simulink model "VSC_GF_2bus_nonlinear"  (R2021b)
settings: Solver=ode45  StartTime=0.0  StopTime=Tsim  FixedStep=10e-6  RelTol=1e-6  EnableMultiTasking=on
values from neighbouring files (symbols this model uses):
  angle_g1_fnl = 0.0    (= 0)    [params_pu.m]
  angle_g1_init = 0.0    (= 0)    [params_pu.m]
  Cac_n1 = 0.15/wb_n1    (= 0.000477464829276)    [params_pu.m]
  k_droop_u_n1 = (0.02/0.3)*(sqrt(2)/sqrt(3))    [params_pu.m]
  ki_pll1 = kp_pll1/tau_pll_n1    [params_pu.m]
  ki_vac_n1 = 42.05*(Vb_n1/Ib_n1)    (= 7.28000181818)    [params_pu.m]
  kp_pll1 = xi_pll_n1*2*omega_pll_n1/(sqrt(2)/sqrt(3))    [params_pu.m]
  kp_vac_n1 = 4.789*(Vb_n1/Ib_n1)    (= 0.829106509091)    [params_pu.m]
  Lc_n1 = 0.15/wb_n1    (= 0.000477464829276)    [params_pu.m]
  Lg_n1 = Xg_n1/wb_n1    [params_pu.m]
  Lg_n2 = imag(Zg_n2)/wb_n1    [params_pu.m]
  magnitud_delay = 1e-5    (= 1e-05)    [params_pu.m]
  P_ref_n1 = 0.5    [params_pu.m]
  plots_step = 10e-6    (= 1e-05)    [params_pu.m]
  Q_ref_n1 = 0.1    [params_pu.m]
  Rac_n1 = 1/(3*10*wb_n1*Cac_n1)    (= 0.222222222222)    [params_pu.m]
  Rg_n1 = Rg_n1/Zb_n1    [params_pu.m]
  Rg_n2 = real(Zg_n2)    [params_pu.m]
  Rseries_n1 = 5e-4/Zb_n1    (= 0.00288804872926)    [params_pu.m]
  T_stp = Tsim/2    (= 2)    [params_pu.m]
  tau_droop_f = 1/50    (= 0.02)    [params_pu.m]
  tau_droop_u = 1/50    (= 0.02)    [params_pu.m]
  tau_ig = 0.1e-3    (= 0.0001)    [params_pu.m]
  tau_u = 0.1e-3    (= 0.0001)    [params_pu.m]
  Vb_dc_n1 = 2e3    (= 2000)    [params_pu.m]
  Vb_n1 = 0.69e3    (= 690)    [params_pu.m]
  Vdcref_n1 = Vb_dc_n1    (= 2000)    [params_pu.m]
  Vpeak_g1_fnl = 0.98*(sqrt(2)/sqrt(3))    [params_pu.m]
  Vpeak_g1_init = 1*(sqrt(2)/sqrt(3))    [params_pu.m]
  Vpeak_n1 = Vb_n1/sqrt(3)*sqrt(2)    [params_pu.m]
  wb_n1 = 2*pi*fb_n1    (= 314.159265359)    [params_pu.m]
undefined symbols (not defined in the file or in its folder): Cac, DRload, Ib_vsc, is_dc0, is_qc0, k_droop_f, ki_s, ki_vac, kp_s, kp_vac, Lc, Lf, Ltr, P, Rac, Rc, Rtr, Sb, T_load, tstep, u_dc0, u_q0, u_qc0, Vb_vsc, vc_dc0, vc_qc0, wb, Zb
libraries: spsSeriesRLCBranchLib x42, spsParallelRLCBranchLib x21, spsControlledVoltageSourceLib x14, spsCurrentMeasurementLib x14, spsGroundLib x10, slpidlib x9, spsVoltageMeasurementLib x6, spsThreePhaseVIMeasurementLib x2, spsPower3phInstantaneousLib x2, spsThreePhaseBreakerLib x2, spsControlledCurrentSourceLib x2, eeTransforms x1
(part 1 of 3)
settings Model: ExtModeTrigDuration=100  Creator=Enric  LastModifiedBy=CITCEA
settings SolverCC: SolverJacobianMethodControl=FullPerturbation  AlgebraicLoopSolver=TrustRegion
settings DataIOCC: LimitDataPoints=on  SaveOutput=off  ReturnWorkspaceOutputs=off  StateSaveName=tmp_raccel_xout  SignalLoggingName=tmp_raccel_logsout
settings OptimizationCC: EfficientMapNaN2IntZero=off  LifeSpan=inf
settings DebuggingCC: AllowSymbolicDim=off  SFUnexpectedBacktrackingDiag=warning  SFNoUnconditionalDefaultTransitionDiag=warning  SFExecutionAtInitializationDiag=none  SFMachineParentedDataDiag=warning  ArithmeticOperatorsInVariantConditions=warning
settings HardwareCC: TargetBitPerPointer=64  TargetBitPerSizeT=64  TargetBitPerPtrDiffT=64  TargetLongLongMode=on  TargetIntDivRoundTo=Zero  TargetEndianess=LittleEndian  TargetWordSize=64  TargetHWDeviceType=MATLAB Host  ProdEqTarget=off
settings ModelReferenceCC: PropagateSignalLabelsOutOfModel=off
settings SFSimCC: SimUseLocalCustomCode=off  CustomCodeUndefinedFunction=UseInterfaceOnly
settings RTWCC: SystemTargetFile=raccel.tlc  TemplateMakefile=raccel_default_tmf  RTWVerbose=off  RTWUseLocalCustomCode=off  RTWUseSimCustomCode=on
settings CodeAppCC: GenerateComments=off  MaxIdLength=128  MangleLength=10  SimulinkBlockComments=off
settings RaccelTargetCC: ENABLE_SLEXEC_SSBRIDGE=0  RTWCAPISignals=off  RTWCAPIParams=on  RTWCAPIRootIO=off
settings ConfigComp: CovMetricSettings=dw  CovSaveCumulativeToWorkspaceVar=on  CovSaveSingleToWorkspaceVar=on  CovExternalEMLEnable=off
settings SimscapeCC: SimscapeNormalizeSystem=off

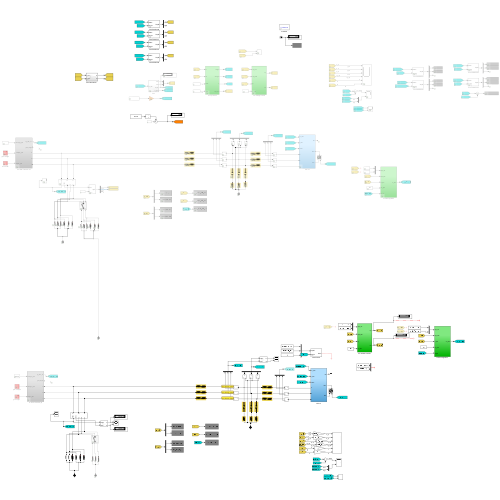
[thumbnail: Simulink's stored preview of the top-level diagram]
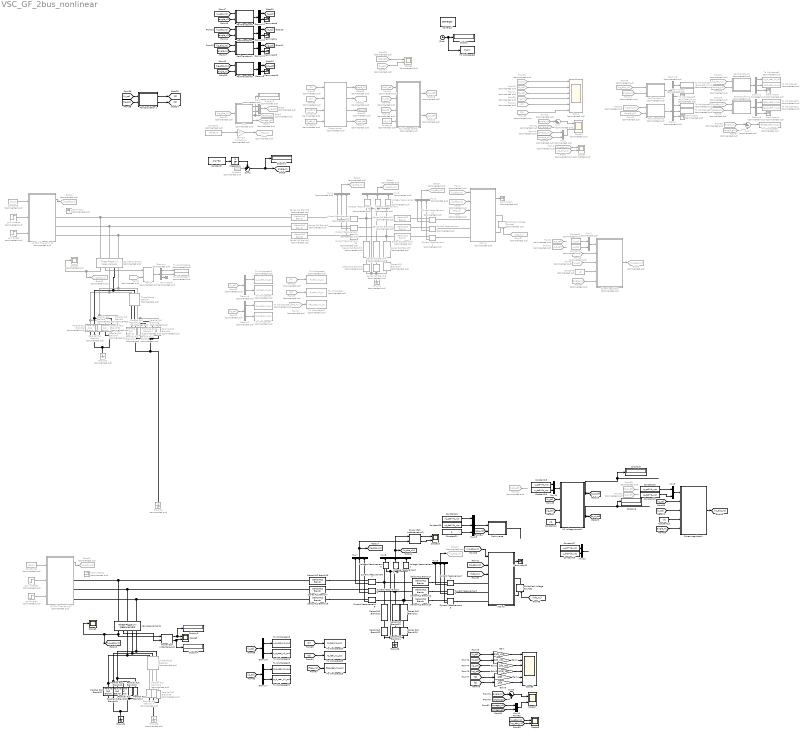
== system VSC_GF_2bus_nonlinear ==
  AC Grid Thevenin g1 : Subsystem  Commented=on
  AC Grid Thevenin g2 : Subsystem  Commented=on
  AC voltage control : Subsystem  Commented=on
  AC voltage control1 : Subsystem
  Clock : Clock
  Constant : Constant  Commented=on  Value=-pi/2
  Constant1 : Constant  Commented=on  Value=Vdcref_n1
  Constant10 : Constant  Value=is_qc0*Ib_vsc
  Constant11 : Constant  Commented=on  Value=wb_n1
  Constant12 : Constant  Value=wb
  Constant13 : Constant  Value=is_dc0*Ib_vsc
  Constant14 : Constant  Value=wb
  Constant15 : Constant  Value=u_qc0*Vb_vsc
  Constant16 : Constant  Value=u_dc0*Vb_vsc
  Constant17 : Constant  Value=u_qc0*Vb_vsc
  Constant18 : Constant  Value=u_dc0*Vb_vsc
  Constant19 : Constant  Value=vc_qc0*Vb_vsc
  Constant2 : Constant  Commented=on  Value=is_qc0
  Constant20 : Constant  Value=vc_dc0*Vb_vsc
  Constant21 : Constant  Value=0
  Constant3 : Constant  Commented=on  Value=P_ref_n1
  Constant4 : Constant  Commented=on  Value=wb_n1
  Constant5 : Constant  Commented=on  Value=wb_n1
  Constant6 : Constant  Commented=on  Value=wb
  Constant7 : Constant  Commented=on  Value=Q_ref_n1
  Constant8 : Constant  Commented=on  Value=is_dc0
  Constant9 : Constant  Value=2*pi*50
  Controlled Voltage Source1 : spsControlledVoltageSourceLib/Controlled Voltage Source  Commented=on  Initialize=off  Source_Type=DC  Amplitude=Vdcref_n1  Phase=0  Frequency=0  Measurements=None
  Controlled Voltage Source2 : spsControlledVoltageSourceLib/Controlled Voltage Source  Initialize=off  Source_Type=DC  Amplitude=Vdcref_n1  Phase=0  Frequency=0  Measurements=None
  Current Measurement{1..2,10,20..21,25} (6 alike) : spsCurrentMeasurementLib/Current Measurement  Commented=on  PhasorSimulation=off  OutputType=Complex  PSBequivalent=0
  Current Measurement{3..8} (6 alike) : spsCurrentMeasurementLib/Current Measurement  PhasorSimulation=off  OutputType=Complex  PSBequivalent=0
  Current regulator : Subsystem  Commented=on
  Current regulator1 : Subsystem
  Demux{,2,4,6,8} (5 alike) : Demux  Commented=on  Outputs=3
  Demux1 : Demux  Commented=on  Outputs=2
  Demux{5,7,9..11,13} (6 alike) : Demux  Outputs=2
  Demux3 : Demux  Commented=on  Outputs=2
  Display{,1,3..6} (6 alike) : Display
  Display2 : Display  Commented=on
  Droop control : Subsystem  Commented=on
  From : From  Commented=on  GotoTag=Vdc_n1
  From1 : From  Commented=on  GotoTag=vc_abc_n1
  From{10,22,34,56} (4 alike) : From  Commented=on  GotoTag=angle_g1
  From{3,11,23,35,52} (5 alike) : From  Commented=on  GotoTag=angle_n1  TagVisibility=global
  From12 : From  Commented=on  GotoTag=P
  From15 : From  Commented=on  GotoTag=is_qd
  From18 : From  Commented=on  GotoTag=is_qd
  From19 : From  Commented=on  GotoTag=is_d_ref
  From2 : From  Commented=on  GotoTag=theta_g
  From{8,20,30,44,46} (5 alike) : From  Commented=on  GotoTag=u_qd
  From21 : From  Commented=on  GotoTag=ig_qd
  From24 : From  Commented=on  GotoTag=P
  From25 : From  Commented=on  GotoTag=Q
  From26 : From  Commented=on  GotoTag=ig_abc_n1
  From27 : From  Commented=on  GotoTag=is_qd
  From28 : From  Commented=on  GotoTag=P
  From29 : From  Commented=on  GotoTag=Q
  From{7,31..32,43} (4 alike) : From  Commented=on  GotoTag=vg_abc_n1
  From33 : From  Commented=on  GotoTag=vg_qd
  From37 : From  Commented=on  GotoTag=Vdc_n1
  From39 : From  Commented=on  GotoTag=vqd_ref
  From4 : From  Commented=on  GotoTag=freq_n1
  From40 : From  Commented=on  GotoTag=omega_g1
  From41 : From  Commented=on  GotoTag=omega_n1
  From49 : From  Commented=on  GotoTag=ig_qd
  From5 : From  Commented=on  GotoTag=is_q_ref
  From51 : From  Commented=on  GotoTag=ig_abc_n1
  From54 : From  Commented=on  GotoTag=vqd_ref
  From55 : From  Commented=on  GotoTag=Q
  From6 : From  Commented=on  GotoTag=u_abc_n1
  From60 : From  Commented=on  GotoTag=is_d_ref
  From61 : From  Commented=on  GotoTag=vqd_ref
  From68 : From  Commented=on  GotoTag=is_q_ref
  From9 : From  Commented=on  GotoTag=is_abc_n1
  Gain : Gain  Gain=1/Vb_vsc
  Gain1 : Gain  Gain=1/Ib_vsc
  Gain10 : Gain  Commented=on  Gain=1/Vb_dc_n1
  Gain2 : Gain  Gain=1/Ib_vsc
  Gain3 : Gain  Gain=1/Vb_vsc
  Gain4 : Gain  Gain=1/Sb
  Gain5 : Gain  Gain=1/Sb
  Goto : Goto  Commented=on  GotoTag=Vdc_n1
  Goto1 : Goto  Commented=on  GotoTag=u_abc_n1
  Goto12 : Goto  Commented=on  GotoTag=vg_abc_n1
  Goto16 : Goto  Commented=on  GotoTag=vg_abc_n1
  Goto18 : Goto  Commented=on  GotoTag=is_q_ref
  Goto19 : Goto  Commented=on  GotoTag=is_d_ref
  Goto2 : Goto  Commented=on  GotoTag=vg_abc_n1
  Goto21 : Goto  Commented=on  GotoTag=omega_n1
  Goto22 : Goto  Commented=on  GotoTag=freq_n1
  Goto25 : Goto  Commented=on  GotoTag=vqd_ref
  Goto27 : Goto  Commented=on  GotoTag=is_abc_n1
  Goto3 : Goto  Commented=on  GotoTag=ig_abc_n1
  Goto4 : Goto  Commented=on  GotoTag=angle_g1
  Goto59 : Goto  Commented=on  GotoTag=angle_n1
  Goto6 : Goto  Commented=on  GotoTag=vc_abc_n1
  Goto7 : Goto  Commented=on  GotoTag=omega_g1
  Goto8 : Goto  Commented=on  GotoTag=vg_qd
  Goto9 : Goto  Commented=on  GotoTag=is_abc_n1
  Ground{,1..2,5} (4 alike) : spsGroundLib/Ground  Commented=on  LConnTagsString=a
  Ground3 : spsGroundLib/Ground  LConnTagsString=a
  Ground4 : spsGroundLib/Ground  LConnTagsString=a
  Icg measurement : spsThreePhaseVIMeasurementLib/Three-Phase V-I Measurement  Commented=on  VoltageMeasurement=phase-to-ground  SetLabelV=off  LabelV=Uabc  Vpu=off  VpuLL=off  CurrentMeasurement=yes  SetLabelI=off  LabelI=Id  Ipu=off  Pbase=100e6  Vbase=500e3  OutputType=Complex  PhasorSimulation=off  PSBequivalent=0
  Icg measurement1 : spsThreePhaseVIMeasurementLib/Three-Phase V-I Measurement  VoltageMeasurement=phase-to-ground  SetLabelV=off  LabelV=Uabc  Vpu=off  VpuLL=off  CurrentMeasurement=yes  SetLabelI=off  LabelI=Id  Ipu=off  Pbase=100e6  Vbase=500e3  OutputType=Complex  PhasorSimulation=off  PSBequivalent=0
  Integrator1 : Integrator
  Mux : Mux  Commented=on  Inputs=2
  Mux1 : Mux  Commented=on  Inputs=2
  Mux{3,10..12} (4 alike) : Mux  Inputs=2
  Mux{7..9,13} (4 alike) : Mux  Inputs=3
  Mux2 : Mux  Commented=on  Inputs=2
  Mux4 : Mux  Commented=on  Inputs=3
  Mux5 : Mux  Commented=on  Inputs=3
  Mux6 : Mux  Commented=on  Inputs=3
  PLL : Subsystem  Commented=on
  PQ Calculation 1 : Subsystem
  Parallel RLC Branch{1..3,7..9} (6 alike) : spsParallelRLCBranchLib/Parallel RLC Branch  Commented=on  LConnTagsString=a  RConnTagsString=__new0  BranchType=L  Resistance=P.R  Inductance=T_load.X/wb  SetiL0=off  InitialCurrent=ini.Ia  Capacitance=1e-6  Setx0=off  InitialVoltage=0  Measurements=None
  Parallel RLC Branch10 : spsParallelRLCBranchLib/Parallel RLC Branch  Commented=on  LConnTagsString=a  RConnTagsString=__new0  BranchType=R  Resistance=T_load.R + DRload  Inductance=3.333/2/pi/60  SetiL0=off  InitialCurrent=ini.Ia  Capacitance=1e-6  Setx0=off  InitialVoltage=0  Measurements=None
  Parallel RLC Branch11 : spsParallelRLCBranchLib/Parallel RLC Branch  Commented=on  LConnTagsString=a  RConnTagsString=__new0  BranchType=R  Resistance=T_load.R + DRload  Inductance=1.1111  SetiL0=off  InitialCurrent=ini.Ia  Capacitance=1e-6  Setx0=off  InitialVoltage=0  Measurements=None
  Parallel RLC Branch12 : spsParallelRLCBranchLib/Parallel RLC Branch  Commented=on  LConnTagsString=a  RConnTagsString=__new0  BranchType=R  Resistance=T_load.R + DRload  Inductance=1.1111  SetiL0=off  InitialCurrent=ini.Ia  Capacitance=1e-6  Setx0=off  InitialVoltage=0  Measurements=None
  Parallel RLC Branch13 : spsParallelRLCBranchLib/Parallel RLC Branch  LConnTagsString=a  RConnTagsString=__new0  BranchType=L  Resistance=P.R  Inductance=T_load.X/wb*Zb  SetiL0=off  InitialCurrent=ini.Ia  Capacitance=1e-6  Setx0=off  InitialVoltage=0  Measurements=None
  Parallel RLC Branch14 : spsParallelRLCBranchLib/Parallel RLC Branch  Commented=on  LConnTagsString=a  RConnTagsString=__new0  BranchType=R  Resistance=(T_load.R/0.01)*Zb  Inductance=1.1111  SetiL0=off  InitialCurrent=ini.Ia  Capacitance=1e-6  Setx0=off  InitialVoltage=0  Measurements=None
  Parallel RLC Branch15 : spsParallelRLCBranchLib/Parallel RLC Branch  Commented=on  LConnTagsString=a  RConnTagsString=__new0  BranchType=R  Resistance=(T_load.R/0.01)*Zb  Inductance=1.1111  SetiL0=off  InitialCurrent=ini.Ia  Capacitance=1e-6  Setx0=off  InitialVoltage=0  Measurements=None
  Parallel RLC Branch16 : spsParallelRLCBranchLib/Parallel RLC Branch  Commented=on  LConnTagsString=a  RConnTagsString=__new0  BranchType=R  Resistance=(T_load.R/0.01)*Zb  Inductance=1.1111  SetiL0=off  InitialCurrent=ini.Ia  Capacitance=1e-6  Setx0=off  InitialVoltage=0  Measurements=None
  Parallel RLC Branch17 : spsParallelRLCBranchLib/Parallel RLC Branch  LConnTagsString=a  RConnTagsString=__new0  BranchType=L  Resistance=P.R  Inductance=T_load.X/wb*Zb  SetiL0=off  InitialCurrent=ini.Ia  Capacitance=1e-6  Setx0=off  InitialVoltage=0  Measurements=None
  Parallel RLC Branch18 : spsParallelRLCBranchLib/Parallel RLC Branch  LConnTagsString=a  RConnTagsString=__new0  BranchType=L  Resistance=P.R  Inductance=T_load.X/wb*Zb  SetiL0=off  InitialCurrent=ini.Ia  Capacitance=1e-6  Setx0=off  InitialVoltage=0  Measurements=None
  Parallel RLC Branch19 : spsParallelRLCBranchLib/Parallel RLC Branch  LConnTagsString=a  RConnTagsString=__new0  BranchType=R  Resistance=T_load.R*Zb  Inductance=1.1111  SetiL0=off  InitialCurrent=ini.Ia  Capacitance=1e-6  Setx0=off  InitialVoltage=0  Measurements=None
  Parallel RLC Branch20 : spsParallelRLCBranchLib/Parallel RLC Branch  LConnTagsString=a  RConnTagsString=__new0  BranchType=R  Resistance=T_load.R*Zb  Inductance=1.1111  SetiL0=off  InitialCurrent=ini.Ia  Capacitance=1e-6  Setx0=off  InitialVoltage=0  Measurements=None
  Parallel RLC Branch21 : spsParallelRLCBranchLib/Parallel RLC Branch  LConnTagsString=a  RConnTagsString=__new0  BranchType=R  Resistance=T_load.R*Zb  Inductance=1.1111  SetiL0=off  InitialCurrent=ini.Ia  Capacitance=1e-6  Setx0=off  InitialVoltage=0  Measurements=None
  Parallel RLC Branch4 : spsParallelRLCBranchLib/Parallel RLC Branch  Commented=on  LConnTagsString=a  RConnTagsString=__new0  BranchType=R  Resistance=T_load.R  Inductance=3.333/2/pi/60  SetiL0=off  InitialCurrent=ini.Ia  Capacitance=1e-6  Setx0=off  InitialVoltage=0  Measurements=None
  Parallel RLC Branch5 : spsParallelRLCBranchLib/Parallel RLC Branch  Commented=on  LConnTagsString=a  RConnTagsString=__new0  BranchType=R  Resistance=T_load.R  Inductance=1.1111  SetiL0=off  InitialCurrent=ini.Ia  Capacitance=1e-6  Setx0=off  InitialVoltage=0  Measurements=None
  Parallel RLC Branch6 : spsParallelRLCBranchLib/Parallel RLC Branch  Commented=on  LConnTagsString=a  RConnTagsString=__new0  BranchType=R  Resistance=T_load.R  Inductance=1.1111  SetiL0=off  InitialCurrent=ini.Ia  Capacitance=1e-6  Setx0=off  InitialVoltage=0  Measurements=None
  Park 3 : eeTransforms/Park Transform  Commented=on  AxisAlignment=Q-axis  PowerInvariant=off
  ParkInverse : Subsystem  mask(Gerard){}
      mask help:
      | This block applies the park inverse transfomation from a desired vector.
      | The input Xqd0 refers to the vector in the qd0 frame, and the second input is the angle used in the inverse transformation.
      | The output is the vector in the ABC frame.
      mask Display:
      | port_label('output',1,'Xabc')
      | port_label('input',1,'Xqd0')
      | port_label('input',2,'angle')
  ParkTransform : Subsystem  mask(Gerard){}
      mask help:
      | This block applies the park transfomation from a desired vector.
      | The input Xabc refers to the vector in the ABC frame, and the second input is the angle used in the transformation.
      | The output is the vector in the qd0 frame.
      mask Display:
      | port_label('output',1,'Xqd0')
      | port_label('input',1,'Xabc')
      | port_label('input',2,'angle')
  ParkTransform1 : Subsystem  mask(Gerard){}
      mask help:
      | This block applies the park transfomation from a desired vector.
      | The input Xabc refers to the vector in the ABC frame, and the second input is the angle used in the transformation.
      | The output is the vector in the qd0 frame.
      mask Display:
      | port_label('output',1,'Xqd0')
      | port_label('input',1,'Xabc')
      | port_label('input',2,'angle')
  ParkTransform2 : Subsystem  Commented=on  mask(Gerard){}
      mask help:
      | This block applies the park transfomation from a desired vector.
      | The input Xabc refers to the vector in the ABC frame, and the second input is the angle used in the transformation.
      | The output is the vector in the qd0 frame.
      mask Display:
      | port_label('output',1,'Xqd0')
      | port_label('input',1,'Xabc')
      | port_label('input',2,'angle')
  ParkTransform3 : Subsystem  Commented=on  mask(Gerard){}
      mask help:
      | This block applies the park transfomation from a desired vector.
      | The input Xabc refers to the vector in the ABC frame, and the second input is the angle used in the transformation.
      | The output is the vector in the qd0 frame.
      mask Display:
      | port_label('output',1,'Xqd0')
      | port_label('input',1,'Xabc')
      | port_label('input',2,'angle')
  ParkTransform4 : Subsystem  Commented=on  mask(Gerard){}
      mask help:
      | This block applies the park transfomation from a desired vector.
      | The input Xabc refers to the vector in the ABC frame, and the second input is the angle used in the transformation.
      | The output is the vector in the qd0 frame.
      mask Display:
      | port_label('output',1,'Xqd0')
      | port_label('input',1,'Xabc')
      | port_label('input',2,'angle')
  ParkTransform5 : Subsystem  mask(Gerard){}
      mask help:
      | This block applies the park transfomation from a desired vector.
      | The input Xabc refers to the vector in the ABC frame, and the second input is the angle used in the transformation.
      | The output is the vector in the qd0 frame.
      mask Display:
      | port_label('output',1,'Xqd0')
      | port_label('input',1,'Xabc')
      | port_label('input',2,'angle')
  ParkTransform6 : Subsystem  mask(Gerard){}
      mask help:
      | This block applies the park transfomation from a desired vector.
      | The input Xabc refers to the vector in the ABC frame, and the second input is the angle used in the transformation.
      | The output is the vector in the qd0 frame.
      mask Display:
      | port_label('output',1,'Xqd0')
      | port_label('input',1,'Xabc')
      | port_label('input',2,'angle')
  ParkTransform8 : Subsystem  Commented=on  mask(Gerard){}
      mask help:
      | This block applies the park transfomation from a desired vector.
      | The input Xabc refers to the vector in the ABC frame, and the second input is the angle used in the transformation.
      | The output is the vector in the qd0 frame.
      mask Display:
      | port_label('output',1,'Xqd0')
      | port_label('input',1,'Xabc')
      | port_label('input',2,'angle')
  "Power (3ph, Instantaneous)" : spsPower3phInstantaneousLib/Power (3ph, Instantaneous)
  "Power (3ph, Instantaneous)1" : spsPower3phInstantaneousLib/Power (3ph, Instantaneous)
  Scope : Scope  Commented=on  NumInputPorts=6
  Scope1 : Scope  Commented=on  NumInputPorts=2
  Scope{7..10} (4 alike) : Scope  NumInputPorts=2
  Scope2 : Scope  Commented=on  NumInputPorts=2
  Scope3 : Scope  Commented=on
  Scope4 : Scope  Commented=on  NumInputPorts=2
  Scope5 : Scope
  Scope6 : Scope  NumInputPorts=6
  Series RLC Branch1 : spsSeriesRLCBranchLib/Series RLC Branch  Commented=on  LConnTagsString=__new0  RConnTagsString=__new0  BranchType=RL  Resistance=Rtr  Inductance=Ltr  SetiL0=off  InitialCurrent=0  Capacitance=0  Setx0=off  InitialVoltage=0  Measurements=None
  Series RLC Branch10 : spsSeriesRLCBranchLib/Series RLC Branch  Commented=on  LConnTagsString=__new0  RConnTagsString=__new0  BranchType=R  Resistance=Rac  Inductance=Lf  SetiL0=off  InitialCurrent=0  Capacitance=Cac_n1  Setx0=on  InitialVoltage=vcini_n1  Measurements=None
  Series RLC Branch11 : spsSeriesRLCBranchLib/Series RLC Branch  LConnTagsString=__new0  RConnTagsString=__new0  BranchType=C  Resistance=Rac_n1  Inductance=Lf  SetiL0=off  InitialCurrent=0  Capacitance=Cac/Zb  Setx0=on  InitialVoltage=u_q0*Vb_vsc  Measurements=None
  Series RLC Branch12 : spsSeriesRLCBranchLib/Series RLC Branch  LConnTagsString=__new0  RConnTagsString=__new0  BranchType=RL  Resistance=Rc*Zb  Inductance=Lc*Zb  SetiL0=off  InitialCurrent=0  Capacitance=0  Setx0=off  InitialVoltage=0  Measurements=None
  Series RLC Branch13 : spsSeriesRLCBranchLib/Series RLC Branch  Commented=on  LConnTagsString=__new0  RConnTagsString=__new0  BranchType=RL  Resistance=Rc  Inductance=Lc  SetiL0=off  InitialCurrent=0  Capacitance=0  Setx0=off  InitialVoltage=0  Measurements=None
  Series RLC Branch14 : spsSeriesRLCBranchLib/Series RLC Branch  Commented=on  LConnTagsString=__new0  RConnTagsString=__new0  BranchType=RL  Resistance=Rc  Inductance=Lc  SetiL0=off  InitialCurrent=0  Capacitance=0  Setx0=off  InitialVoltage=0  Measurements=None
  Series RLC Branch15 : spsSeriesRLCBranchLib/Series RLC Branch  Commented=on  LConnTagsString=__new0  RConnTagsString=__new0  BranchType=RL  Resistance=Rc  Inductance=Lc  SetiL0=off  InitialCurrent=0  Capacitance=0  Setx0=off  InitialVoltage=0  Measurements=None
  Series RLC Branch16 : spsSeriesRLCBranchLib/Series RLC Branch  LConnTagsString=__new0  RConnTagsString=__new0  BranchType=RL  Resistance=Rc*Zb  Inductance=Lc*Zb  SetiL0=off  InitialCurrent=0  Capacitance=0  Setx0=off  InitialVoltage=0  Measurements=None
  Series RLC Branch17 : spsSeriesRLCBranchLib/Series RLC Branch  LConnTagsString=__new0  RConnTagsString=__new0  BranchType=RL  Resistance=Rc*Zb  Inductance=Lc*Zb  SetiL0=off  InitialCurrent=0  Capacitance=0  Setx0=off  InitialVoltage=0  Measurements=None
  Series RLC Branch18 : spsSeriesRLCBranchLib/Series RLC Branch  LConnTagsString=__new0  RConnTagsString=__new0  BranchType=RL  Resistance=Rtr*Zb  Inductance=Ltr*Zb  SetiL0=off  InitialCurrent=0  Capacitance=0  Setx0=off  InitialVoltage=0  Measurements=None
  Series RLC Branch19 : spsSeriesRLCBranchLib/Series RLC Branch  LConnTagsString=__new0  RConnTagsString=__new0  BranchType=RL  Resistance=Rtr*Zb  Inductance=Ltr*Zb  SetiL0=off  InitialCurrent=0  Capacitance=0  Setx0=off  InitialVoltage=0  Measurements=None
  Series RLC Branch2 : spsSeriesRLCBranchLib/Series RLC Branch  Commented=on  LConnTagsString=__new0  RConnTagsString=__new0  BranchType=RL  Resistance=Rtr  Inductance=Ltr  SetiL0=off  InitialCurrent=0  Capacitance=0  Setx0=off  InitialVoltage=0  Measurements=None
  Series RLC Branch20 : spsSeriesRLCBranchLib/Series RLC Branch  LConnTagsString=__new0  RConnTagsString=__new0  BranchType=R  Resistance=Rac*Zb  Inductance=Lf  SetiL0=off  InitialCurrent=0  Capacitance=Cac_n1  Setx0=on  InitialVoltage=vcini_n1  Measurements=None
  Series RLC Branch21 : spsSeriesRLCBranchLib/Series RLC Branch  LConnTagsString=__new0  RConnTagsString=__new0  BranchType=C  Resistance=Rac_n1  Inductance=Lf  SetiL0=off  InitialCurrent=0  Capacitance=Cac/Zb  Setx0=on  InitialVoltage=u_q0*Vb_vsc  Measurements=None
  Series RLC Branch22 : spsSeriesRLCBranchLib/Series RLC Branch  LConnTagsString=__new0  RConnTagsString=__new0  BranchType=R  Resistance=Rac*Zb  Inductance=Lf  SetiL0=off  InitialCurrent=0  Capacitance=Cac_n1  Setx0=on  InitialVoltage=vcini_n1  Measurements=None
  Series RLC Branch23 : spsSeriesRLCBranchLib/Series RLC Branch  LConnTagsString=__new0  RConnTagsString=__new0  BranchType=C  Resistance=Rac_n1  Inductance=Lf  SetiL0=off  InitialCurrent=0  Capacitance=Cac/Zb  Setx0=on  InitialVoltage=u_q0*Vb_vsc  Measurements=None
  Series RLC Branch24 : spsSeriesRLCBranchLib/Series RLC Branch  LConnTagsString=__new0  RConnTagsString=__new0  BranchType=R  Resistance=Rac*Zb  Inductance=Lf  SetiL0=off  InitialCurrent=0  Capacitance=Cac_n1  Setx0=on  InitialVoltage=vcini_n1  Measurements=None
  Series RLC Branch3 : spsSeriesRLCBranchLib/Series RLC Branch  Commented=on  LConnTagsString=__new0  RConnTagsString=__new0  BranchType=RL  Resistance=Rtr  Inductance=Ltr  SetiL0=off  InitialCurrent=0  Capacitance=0  Setx0=off  InitialVoltage=0  Measurements=None
  Series RLC Branch4 : spsSeriesRLCBranchLib/Series RLC Branch  Commented=on  LConnTagsString=__new0  RConnTagsString=__new0  BranchType=C  Resistance=Rac_n1  Inductance=Lf  SetiL0=off  InitialCurrent=0  Capacitance=Cac  Setx0=on  InitialVoltage=u_q0  Measurements=None
  Series RLC Branch5 : spsSeriesRLCBranchLib/Series RLC Branch  Commented=on  LConnTagsString=__new0  RConnTagsString=__new0  BranchType=C  Resistance=Rac_n1  Inductance=Lf  SetiL0=off  InitialCurrent=0  Capacitance=Cac  Setx0=on  InitialVoltage=u_q0  Measurements=None
  Series RLC Branch6 : spsSeriesRLCBranchLib/Series RLC Branch  Commented=on  LConnTagsString=__new0  RConnTagsString=__new0  BranchType=R  Resistance=Rac  Inductance=Lf  SetiL0=off  InitialCurrent=0  Capacitance=Cac_n1  Setx0=on  InitialVoltage=vcini_n1  Measurements=None
  Series RLC Branch7 : spsSeriesRLCBranchLib/Series RLC Branch  LConnTagsString=__new0  RConnTagsString=__new0  BranchType=RL  Resistance=Rtr*Zb  Inductance=Ltr*Zb  SetiL0=off  InitialCurrent=0  Capacitance=0  Setx0=off  InitialVoltage=0  Measurements=None
  Series RLC Branch8 : spsSeriesRLCBranchLib/Series RLC Branch  Commented=on  LConnTagsString=__new0  RConnTagsString=__new0  BranchType=R  Resistance=Rac  Inductance=Lf  SetiL0=off  InitialCurrent=0  Capacitance=Cac_n1  Setx0=on  InitialVoltage=vcini_n1  Measurements=None
  Series RLC Branch9 : spsSeriesRLCBranchLib/Series RLC Branch  Commented=on  LConnTagsString=__new0  RConnTagsString=__new0  BranchType=C  Resistance=Rac_n1  Inductance=Lf  SetiL0=off  InitialCurrent=0  Capacitance=Cac  Setx0=on  InitialVoltage=u_q0  Measurements=None
  Sum : Sum  Commented=on  Inputs=|+-
  Sum1 : Sum  Commented=on  Inputs=|+-
  Sum2 : Sum  Inputs=++|
  Sum3 : Sum  Inputs=|+-
  Terminator{,1..3,6..7,9,11} (8 alike) : Terminator  Commented=on
  Terminator{4..5,8,10,12} (5 alike) : Terminator
  Three-Phase Breaker : spsThreePhaseBreakerLib/Three-Phase Breaker  Commented=on  InitialState=open  SwitchA=on  SwitchB=on  SwitchC=on  SwitchTimes=[tstep 1000]  External=off  BreakerResistance=0.0001  SnubberResistance=inf  SnubberCapacitance=inf  Measurements=None
  Three-Phase Breaker1 : spsThreePhaseBreakerLib/Three-Phase Breaker  Commented=on  InitialState=open  SwitchA=on  SwitchB=on  SwitchC=on  SwitchTimes=[tstep 1000]  External=off  BreakerResistance=0.0001  SnubberResistance=inf  SnubberCapacitance=inf  Measurements=None
  To Workspace1 : ToWorkspace  Commented=on  VariableName=ig_d_real_n1_pu  SampleTime=plots_step
  To Workspace10 : ToWorkspace  Commented=on  VariableName=u_q_real_n1_pu  SampleTime=plots_step
  To Workspace11 : ToWorkspace  Commented=on  VariableName=freq_real_n1_pu  SampleTime=plots_step
  To Workspace12 : ToWorkspace  Commented=on  VariableName=igc_d_real_n1_pu  SampleTime=plots_step
  To Workspace13 : ToWorkspace  Commented=on  VariableName=igc_q_real_n1_pu  SampleTime=plots_step
  To Workspace14 : ToWorkspace  Commented=on  VariableName=vgc_q_real_n1_pu  SampleTime=plots_step
  To Workspace15 : ToWorkspace  Commented=on  VariableName=vgc_d_real_n1_pu  SampleTime=plots_step
  To Workspace16 : ToWorkspace  Commented=on  VariableName=icgd_nolin  SampleTime=1e-4
  To Workspace17 : ToWorkspace  Commented=on  VariableName=icgq_nolin  SampleTime=1e-4
  To Workspace18 : ToWorkspace  VariableName=u_q_real_n1_pu1  SampleTime=plots_step
  To Workspace19 : ToWorkspace  VariableName=freq_real_n1_pu1  SampleTime=plots_step
  To Workspace2 : ToWorkspace  VariableName=tnolin  SampleTime=plots_step
  To Workspace22 : ToWorkspace  VariableName=is_d_real_n1_pu1  SampleTime=plots_step
  To Workspace23 : ToWorkspace  VariableName=is_q_real_n1_pu1  SampleTime=plots_step
  To Workspace24 : ToWorkspace  VariableName=P_real_n1_pu1  SampleTime=plots_step
  To Workspace25 : ToWorkspace  VariableName=Q_real_n1_pu1  SampleTime=plots_step
  To Workspace26 : ToWorkspace  VariableName=u_d_real_n1_pu1  SampleTime=plots_step
  To Workspace28 : ToWorkspace  Commented=on  VariableName=vg_q_real_n1_pu  SampleTime=plots_step
  To Workspace29 : ToWorkspace  Commented=on  VariableName=vg_d_real_n1_pu  SampleTime=plots_step
  To Workspace3 : ToWorkspace  Commented=on  VariableName=ig_q_real_n1_pu  SampleTime=plots_step
  To Workspace4 : ToWorkspace  Commented=on  VariableName=is_d_real_n1_pu  SampleTime=plots_step
  To Workspace5 : ToWorkspace  Commented=on  VariableName=is_q_real_n1_pu  SampleTime=plots_step
  To Workspace6 : ToWorkspace  Commented=on  VariableName=P_real_n1_pu  SampleTime=plots_step
  To Workspace7 : ToWorkspace  Commented=on  VariableName=Q_real_n1_pu  SampleTime=plots_step
  To Workspace8 : ToWorkspace  Commented=on  VariableName=u_d_real_n1_pu  SampleTime=plots_step
  To Workspace9 : ToWorkspace  Commented=on  VariableName=etheta_real_n1_pu  SampleTime=plots_step
  VSC n1 : Subsystem  Commented=on
  VSC n2 : Subsystem
  Voltage Measurement1 : spsVoltageMeasurementLib/Voltage Measurement  PhasorSimulation=off  OutputType=Complex  PSBequivalent=0
  Voltage Measurement2 : spsVoltageMeasurementLib/Voltage Measurement  PhasorSimulation=off  OutputType=Complex  PSBequivalent=0
  Voltage Measurement3 : spsVoltageMeasurementLib/Voltage Measurement  Commented=on  PhasorSimulation=off  OutputType=Complex  PSBequivalent=0
  Voltage Measurement4 : spsVoltageMeasurementLib/Voltage Measurement  Commented=on  PhasorSimulation=off  OutputType=Complex  PSBequivalent=0
  Voltage Measurement5 : spsVoltageMeasurementLib/Voltage Measurement  PhasorSimulation=off  OutputType=Complex  PSBequivalent=0
  Voltage Measurement6 : spsVoltageMeasurementLib/Voltage Measurement  Commented=on  PhasorSimulation=off  OutputType=Complex  PSBequivalent=0
  grid angle : Step  Commented=on  Time=T_stp  Before=angle_g1_init  After=angle_g1_fnl  SampleTime=0
  grid angle1 : Step  Commented=on  Time=T_stp  Before=angle_g1_init  After=angle_g1_fnl  SampleTime=0
  grid voltage : Step  Commented=on  Time=T_stp  Before=Vpeak_g1_init  After=Vpeak_g1_fnl  SampleTime=0
  grid voltage1 : Step  Commented=on  Time=T_stp  Before=Vpeak_g1_init  After=Vpeak_g1_fnl  SampleTime=0
  powergui : spspowerguiLib/powergui  Priority=1  SimulationMode=Continuous  SampleTime=1e-5  frequency=60  Iterations=50  frequencyindice=0  Pbase=100e6  ErrMax=1e-4  UnitsV=kV  UnitsW=MW  buscounter=0  FunctionMessages=off  echomessages=off  EnableUseOfTLC=off  CurrentSourceSwitches=off  DisableSnubberDevices=off  DisableRonSwitches=off  DisableVfSwitches=off  DisplayEquations=off  AutomaticDiscreteSolvers=off  SolverType=Tustin  Interpol=off  ExternalGateDelay=off  methode=off  Ts=0  x0status=blocks  SPID=off  SwTol=0  HookPort=off  NonlinearTolerance=1e-4  nMaxIteration=100  ContinueOnMaxIteration=off  RestoreLinks=warning  ResistiveCurrentMeasurement=off  Frange=[0:2:500]  Ylog=off  Xlog=on  ShowGrid=off  save=off  variable=ZData  structure=Vk  ZoomFFT=off  StartTime=2.01  cycles=3  DisplayStyle=1  fundamental=50  FreqAxis=off  MaxFrequency=1000  frequencyindicesteady=1  RmsSteady=1  display=off
  tag scope: angle_n1=global
  wires:
  Voltage Measurement4/1 -> Mux5/2
  Voltage Measurement3/1 -> Mux5/3
  Voltage Measurement6/1 -> Mux5/1
  Clock/1 -> To Workspace2/1, Display/1
  VSC n1/1(idc) -> Terminator7/1
  From8/1 -> Current regulator/3(u_ffw)
  Constant6/1 -> Current regulator/4(w_grid)
  Mux2/1 -> Current regulator/1(iqd_ref)
  From15/1 -> Current regulator/2(iqd_fdb)
  From/1 -> VSC n1/3(Vbus)
  From9/1 -> VSC n1/2(i_abc)
  Current regulator/1(vc_abc) -> Goto6/1
  From1/1 -> VSC n1/1(vc_abc)
  From52/1 -> Current regulator/5(angle)
  Current Measurement1/1 -> Mux6/2
  Current Measurement2/1 -> Mux6/3
  Current Measurement10/1 -> Mux6/1
  [angle_n1] -> ParkTransform/2(angle)
  [is_abc_n1] -> ParkTransform/1(ABC vector)
  [angle_n1] -> ParkTransform1/2(angle)
  [ig_abc_n1] -> ParkTransform1/1(ABC vector)
  ParkTransform1/1(Matrix) -> Demux11/1
  From20/1 -> Scope/1  "u_qd"
  From18/1 -> Scope/2  "is_qd"
  From21/1 -> Scope/3  "ig_qd"
  From25/1 -> Scope/6  "Q"
  From28/1 -> To Workspace6/1
  From29/1 -> To Workspace7/1
  Demux3/2 -> To Workspace8/1
  Demux3/1 -> To Workspace10/1
  From30/1 -> Demux3/1
  From27/1 -> Demux1/1
  Demux1/1 -> To Workspace5/1
  Demux1/2 -> To Workspace4/1
  ParkTransform/1(Matrix) -> Demux10/1
  Demux10/1 -> [is_qd]
  Demux10/2 -> Terminator4/1
  Demux11/2 -> Terminator5/1
  Demux11/1 -> [ig_qd]
  AC voltage control/1(iq*) -> Goto18/1
  Constant4/1 -> AC voltage control/4(w_grid)
  From46/1 -> AC voltage control/2(vqd_fdb)
  Demux13/2 -> Terminator8/1
  Demux13/1 -> [u_qd]
  ParkTransform6/1(Matrix) -> Demux13/1
  [u_abc_n1] -> ParkTransform6/1(ABC vector)
  [angle_n1] -> ParkTransform6/2(angle)
  From49/1 -> AC voltage control/3(Ig)
  Current Measurement21/1 -> Mux4/1
  Current Measurement25/1 -> Mux4/3
  Current Measurement20/1 -> Mux4/2
  From12/1 -> Droop control/1(P)
  From55/1 -> Droop control/2(Q)
  Droop control/1(angle) -> Goto59/1
  Droop control/2(omega) -> Goto21/1
  Droop control/3(f) -> Goto22/1
  Droop control/4(vqd_ref) -> Goto25/1
  From54/1 -> AC voltage control/1(vqd_ref)
  Demux/3 -> Terminator1/1
  ParkTransform8/1(Matrix) -> Demux/1
  Demux/2 -> To Workspace29/1
  Demux/1 -> To Workspace28/1
  From32/1 -> ParkTransform8/1(ABC vector)
  From4/1 -> To Workspace11/1
  AC voltage control/2(id*) -> Goto19/1
  From6/1 -> Scope4/1
  AC Grid Thevenin g1/1(vg_abc_n1) -> Goto2/1
  From7/1 -> Scope4/2
  From23/1 -> Sum/1
  From22/1 -> Sum/2
  Sum/1 -> Scope1/1  "e_theta"
  Constant5/1 -> AC Grid Thevenin g1/1(Omega_grid)
  PLL/1(Vzq) -> Mux/1
  PLL/2(Vzd) -> Mux/2
  Constant3/1 -> Droop control/3(Pref)  "P*"
  Constant7/1 -> Droop control/4(Qref)  "Q*"
  From34/1 -> Sum1/2
  Sum1/1 -> To Workspace9/1
  From31/1 -> PLL/1(u_abc)
  From41/1 -> Mux1/1  "wn1"
  From40/1 -> Mux1/2  "wg1"
  From3/1 -> ParkTransform2/2(angle)
  ParkTransform2/1(Matrix) -> Demux6/1
  Demux6/1 -> To Workspace13/1
  Demux6/2 -> To Workspace12/1
  Demux6/3 -> Terminator6/1
  From10/1 -> ParkTransform8/2(angle)
  From35/1 -> Sum1/1
  grid voltage/1 -> AC Grid Thevenin g1/2(voltage_grid)
  grid angle/1 -> AC Grid Thevenin g1/3(angle_grid)
  From43/1 -> ParkTransform4/1(ABC vector)
  From11/1 -> ParkTransform4/2(angle)
  Demux8/2 -> To Workspace15/1
  Demux8/1 -> To Workspace14/1
  ParkTransform4/1(Matrix) -> Demux8/1
  Demux8/3 -> Terminator2/1
  [u_qd] -> PQ Calculation 1/1(u_qd)
  [ig_qd] -> PQ Calculation 1/2(ig_qd)
  Mux/1 -> Goto8/1
  From26/1 -> ParkTransform2/1(ABC vector)
  From33/1 -> Scope/4  "vg_qd"
  Mux1/1 -> Scope1/2
  Constant1/1 -> Gain10/1
  From39/1 -> Scope2/1
  From44/1 -> Scope2/2
  From24/1 -> Scope/5  "P"
  PQ Calculation 1/1(P) -> [P]
  PQ Calculation 1/2(Q) -> [Q]
  From51/1 -> ParkTransform3/1(ABC vector)
  Demux2/3 -> Terminator3/1
  ParkTransform3/1(Matrix) -> Demux2/1
  Demux2/2 -> To Workspace1/1
  Demux2/1 -> To Workspace3/1
  From56/1 -> ParkTransform3/2(angle)
  Mux5/1 -> Goto1/1
  Mux4/1 -> Goto3/1
  Mux6/1 -> Goto9/1
  From37/1 -> Controlled Voltage Source1/1
  Gain10/1 -> Goto/1
  PLL/3(angle) -> Display2/1, Goto4/1
  PLL/4(w_grid) -> Goto7/1
  Icg measurement/2 -> Park 3/1
  From2/1 -> Park 3/2
  Park 3/1 -> Demux4/1
  Demux4/2 -> To Workspace17/1  "Icg_q"
  Demux4/3 -> Terminator9/1
  Demux4/1 -> To Workspace16/1  "Icg_d"
  From19/1 -> ?
  From5/1 -> ?
  Constant2/1 -> Mux2/1
  Constant8/1 -> Mux2/2
  Constant9/1 -> Integrator1/1
  Integrator1/1 -> Sum2/1
  Constant/1 -> Sum2/2
  Sum2/1 -> Display1/1, [angle_n1]
  Icg measurement/1 -> Scope3/1, Goto12/1
  [angle_n1] -> ParkTransform5/2(angle)
  Demux5/1 -> [vg_qd]
  ParkTransform5/1(Matrix) -> Demux5/1
  Demux5/2 -> Terminator10/1
  [vg_abc_n1] -> ParkTransform5/1(ABC vector)
  Icg measurement1/1 -> Scope5/1, [vg_abc_n1], "Power (3ph, Instantaneous)"/1
  From68/1 -> ?
  Icg measurement1/2 -> "Power (3ph, Instantaneous)"/2
  AC voltage control1/1(iq*) -> Display5/1, [is_q_ref]
  From60/1 -> ?
  ParkInverse/1(Matrix) -> ?
  [Vdc_n1] -> VSC n2/3(Vbus)
  [is_qd] -> Current regulator1/2(iqd_fdb)
  Current regulator1/1(vc_abc) -> [vc_abc_n1]
  Voltage Measurement2/1 -> Mux8/2
  Mux3/1 -> Current regulator1/1(iqd_ref)
  Current Measurement8/1 -> Mux7/3
  Mux7/1 -> "Power (3ph, Instantaneous)1"/2, [ig_abc_n1]
  Voltage Measurement1/1 -> Mux8/3
  [u_qd] -> Current regulator1/3(u_ffw)
  [is_qd] -> Demux7/1
  Demux9/1 -> To Workspace18/1
  grid voltage1/1 -> AC Grid Thevenin g2/2(voltage_grid)
  Mux8/1 -> "Power (3ph, Instantaneous)1"/1, [u_abc_n1]
  [u_qd] -> Demux9/1
  Constant11/1 -> AC Grid Thevenin g2/1(Omega_grid)
  [Vdc_n1] -> Controlled Voltage Source2/1
  Demux9/2 -> To Workspace26/1
  grid angle1/1 -> AC Grid Thevenin g2/3(angle_grid)
  Current Measurement7/1 -> Mux7/1
  Current Measurement6/1 -> Mux7/2
  [is_abc_n1] -> VSC n2/2(i_abc)
  AC Grid Thevenin g2/1(vg_abc_n1) -> Goto16/1
  Demux7/1 -> To Workspace23/1
  Voltage Measurement5/1 -> Mux8/1
  Mux9/1 -> Goto27/1
  Current Measurement3/1 -> Mux9/2
  Demux7/2 -> To Workspace22/1
  Current Measurement4/1 -> Mux9/1
  [Q] -> To Workspace25/1
  [P] -> To Workspace24/1
  [angle_n1] -> Current regulator1/5(angle)
  Constant12/1 -> Current regulator1/4(w_grid)
  Current Measurement5/1 -> Mux9/3
  VSC n2/1(idc) -> Terminator12/1
  [freq_n1] -> To Workspace19/1
  [P] -> Gain4/1  "P"
  [omega_g1] -> Mux10/2  "wg1"
  [is_qd] -> Gain1/1  "is_qd"
  Mux10/1 -> Scope7/2
  [u_abc_n1] -> Scope8/1
  [angle_g1] -> Sum3/2
  [omega_n1] -> Mux10/1  "wn1"
  [vg_abc_n1] -> Scope8/2
  [Q] -> Gain5/1  "Q"
  [ig_qd] -> Gain2/1  "ig_qd"
  [angle_n1] -> Sum3/1
  [vg_qd] -> Gain3/1  "vg_qd"
  Sum3/1 -> Scope7/1  "e_theta"
  [u_qd] -> Gain/1  "u_qd"
  Gain2/1 -> Scope6/3  "ig_qd"
  Gain1/1 -> Scope6/2  "is_qd"
  Gain/1 -> Scope6/1  "u_qd"
  Gain3/1 -> Scope6/4  "vg_qd"
  Gain4/1 -> Scope6/5  "P"
  Gain5/1 -> Scope6/6  "Q"
  "Power (3ph, Instantaneous)"/1 -> Display3/1, Scope9/1
  "Power (3ph, Instantaneous)"/2 -> Display4/1, Scope9/2
  [ig_qd] -> AC voltage control1/3(Ig)
  Constant14/1 -> AC voltage control1/4(w_grid)
  AC voltage control1/2(id*) -> Display6/1, [is_d_ref]
  [u_qd] -> AC voltage control1/2(vqd_fdb)
  From61/1 -> ?
  Mux11/1 -> AC voltage control1/1(vqd_ref)
  Constant15/1 -> Mux11/1
  Constant16/1 -> Mux11/2
  "Power (3ph, Instantaneous)1"/1 -> Scope10/1
  "Power (3ph, Instantaneous)1"/2 -> Scope10/2
  Constant10/1 -> Mux3/1
  Constant13/1 -> Mux3/2
  Constant17/1 -> Mux12/1
  Mux12/1 -> ?
  Constant18/1 -> Mux12/2
  Mux13/1 -> ParkInverse/1(ABC vector)
  Constant19/1 -> Mux13/1
  [angle_n1] -> ParkInverse/2(angle)
  Constant21/1 -> Mux13/3
  Constant20/1 -> Mux13/2
  [vc_abc_n1] -> VSC n2/1(vc_abc)
  connections:
  Current Measurement2/LConn1 -- VSC n1/LConn3
  VSC n1/LConn1 -- Current Measurement10/LConn1
  Current Measurement1/LConn1 -- VSC n1/LConn2
  Controlled Voltage Source1/RConn1 -- VSC n1/RConn1
  VSC n1/RConn2 -- Controlled Voltage Source1/LConn1
  Series RLC Branch15/LConn1 -- Series RLC Branch5/LConn1 -- Current Measurement21/LConn1 -- Voltage Measurement6/LConn1
  Voltage Measurement6/LConn2 -- Voltage Measurement3/LConn2 -- Voltage Measurement4/LConn2 -- Series RLC Branch8/RConn1 -- Ground/LConn1 -- Series RLC Branch10/RConn1 -- Series RLC Branch6/RConn1
  Current Measurement10/RConn1 -- Series RLC Branch15/RConn1
  Current Measurement1/RConn1 -- Series RLC Branch13/RConn1
  Current Measurement2/RConn1 -- Series RLC Branch14/RConn1
  Series RLC Branch14/LConn1 -- Current Measurement25/LConn1 -- Series RLC Branch9/LConn1 -- Voltage Measurement3/LConn1
  Series RLC Branch13/LConn1 -- Current Measurement20/LConn1 -- Series RLC Branch4/LConn1 -- Voltage Measurement4/LConn1
  Current Measurement25/RConn1 -- Series RLC Branch2/RConn1
  Current Measurement20/RConn1 -- Series RLC Branch1/RConn1
  Current Measurement21/RConn1 -- Series RLC Branch3/RConn1
  Series RLC Branch2/LConn1 -- Icg measurement/LConn3 -- AC Grid Thevenin g1/RConn3
  Series RLC Branch1/LConn1 -- Icg measurement/LConn2 -- AC Grid Thevenin g1/RConn2
  Series RLC Branch3/LConn1 -- Icg measurement/LConn1 -- AC Grid Thevenin g1/RConn1
  Series RLC Branch6/LConn1 -- Series RLC Branch5/RConn1
  Series RLC Branch8/LConn1 -- Series RLC Branch4/RConn1
  Series RLC Branch10/LConn1 -- Series RLC Branch9/RConn1
  Icg measurement/RConn1 -- Parallel RLC Branch3/LConn1 -- Parallel RLC Branch6/LConn1 -- Three-Phase Breaker/RConn1
  Three-Phase Breaker/RConn2 -- Icg measurement/RConn2 -- Parallel RLC Branch1/LConn1 -- Parallel RLC Branch4/LConn1
  Icg measurement/RConn3 -- Parallel RLC Branch2/LConn1 -- Parallel RLC Branch5/LConn1 -- Three-Phase Breaker/RConn3
  Parallel RLC Branch11/LConn1 -- Parallel RLC Branch8/LConn1 -- Three-Phase Breaker/LConn3
  Parallel RLC Branch10/LConn1 -- Parallel RLC Branch7/LConn1 -- Three-Phase Breaker/LConn2
  Parallel RLC Branch12/LConn1 -- Parallel RLC Branch9/LConn1 -- Three-Phase Breaker/LConn1
  Parallel RLC Branch5/RConn1 -- Parallel RLC Branch6/RConn1 -- Parallel RLC Branch4/RConn1 -- Ground1/LConn1 -- Parallel RLC Branch1/RConn1 -- Parallel RLC Branch2/RConn1 -- Parallel RLC Branch3/RConn1
  Parallel RLC Branch11/RConn1 -- Ground2/LConn1 -- Parallel RLC Branch7/RConn1 -- Parallel RLC Branch8/RConn1 -- Parallel RLC Branch9/RConn1 -- Parallel RLC Branch12/RConn1 -- Parallel RLC Branch10/RConn1
  Parallel RLC Branch21/LConn1 -- Parallel RLC Branch18/LConn1 -- Icg measurement1/RConn1 -- Three-Phase Breaker1/RConn1
  Parallel RLC Branch21/RConn1 -- Parallel RLC Branch20/RConn1 -- Parallel RLC Branch19/RConn1 -- Ground4/LConn1 -- Parallel RLC Branch18/RConn1 -- Parallel RLC Branch13/RConn1 -- Parallel RLC Branch17/RConn1
  Icg measurement1/RConn2 -- Three-Phase Breaker1/RConn2 -- Parallel RLC Branch19/LConn1 -- Parallel RLC Branch13/LConn1
  Parallel RLC Branch15/RConn1 -- Parallel RLC Branch16/RConn1 -- Parallel RLC Branch14/RConn1 -- Ground5/LConn1
  Parallel RLC Branch15/LConn1 -- Three-Phase Breaker1/LConn3
  Parallel RLC Branch16/LConn1 -- Three-Phase Breaker1/LConn2
  Series RLC Branch22/RConn1 -- Voltage Measurement5/LConn2 -- Voltage Measurement1/LConn2 -- Voltage Measurement2/LConn2 -- Series RLC Branch24/RConn1 -- Ground3/LConn1 -- Series RLC Branch20/RConn1
  AC Grid Thevenin g2/RConn2 -- Series RLC Branch7/RConn1 -- Icg measurement1/LConn2
  AC Grid Thevenin g2/RConn3 -- Series RLC Branch18/RConn1 -- Icg measurement1/LConn3
  Parallel RLC Branch14/LConn1 -- Three-Phase Breaker1/LConn1
  Three-Phase Breaker1/RConn3 -- Parallel RLC Branch20/LConn1 -- Parallel RLC Branch17/LConn1 -- Icg measurement1/RConn3
  Voltage Measurement2/LConn1 -- Series RLC Branch12/RConn1 -- Series RLC Branch23/LConn1 -- Current Measurement6/LConn1
  AC Grid Thevenin g2/RConn1 -- Series RLC Branch19/RConn1 -- Icg measurement1/LConn1
  Voltage Measurement1/LConn1 -- Series RLC Branch16/RConn1 -- Series RLC Branch11/LConn1 -- Current Measurement8/LConn1
  Voltage Measurement5/LConn1 -- Series RLC Branch17/RConn1 -- Series RLC Branch21/LConn1 -- Current Measurement7/LConn1
  Series RLC Branch22/LConn1 -- Series RLC Branch21/RConn1
  Series RLC Branch7/LConn1 -- Current Measurement6/RConn1
  VSC n2/RConn2 -- Controlled Voltage Source2/LConn1
  Controlled Voltage Source2/RConn1 -- VSC n2/RConn1
  VSC n2/LConn1 -- Current Measurement4/LConn1
  Series RLC Branch18/LConn1 -- Current Measurement8/RConn1
  Series RLC Branch16/LConn1 -- Current Measurement5/RConn1
  Series RLC Branch12/LConn1 -- Current Measurement3/RConn1
  Current Measurement3/LConn1 -- VSC n2/LConn2
  Series RLC Branch19/LConn1 -- Current Measurement7/RConn1
  Series RLC Branch17/LConn1 -- Current Measurement4/RConn1
  Current Measurement5/LConn1 -- VSC n2/LConn3
  Series RLC Branch20/LConn1 -- Series RLC Branch11/RConn1
  Series RLC Branch24/LConn1 -- Series RLC Branch23/RConn1

== system VSC_GF_2bus_nonlinear/AC Grid Thevenin g1 ==
  note: Grid Thevenin
  Omega_grid : Inport
  voltage_grid : Inport  Port=2
  angle_grid : Inport  Port=3
  Controlled Voltage Source3 : spsControlledVoltageSourceLib/Controlled Voltage Source  Initialize=on  Source_Type=AC  Amplitude=0  Phase=0  Frequency=0  Measurements=None
  Controlled Voltage Source4 : spsControlledVoltageSourceLib/Controlled Voltage Source  Initialize=on  Source_Type=AC  Amplitude=0  Phase=0  Frequency=0  Measurements=None
  Controlled Voltage Source5 : spsControlledVoltageSourceLib/Controlled Voltage Source  Initialize=on  Source_Type=AC  Amplitude=0  Phase=0  Frequency=0  Measurements=None
  Grid : Subsystem
  Ground : spsGroundLib/Ground  LConnTagsString=a
  Mux5 : Mux  Inputs=3
  Series RLC Branch1 : spsSeriesRLCBranchLib/Series RLC Branch  LConnTagsString=__new0  RConnTagsString=__new0  BranchType=RL  Resistance=Rg_n2  Inductance=Lg_n2  SetiL0=off  InitialCurrent=0  Capacitance=0  Setx0=off  InitialVoltage=0  Measurements=None
  Series RLC Branch10 : spsSeriesRLCBranchLib/Series RLC Branch  LConnTagsString=__new0  RConnTagsString=__new0  BranchType=RL  Resistance=Rg_n1  Inductance=Lg_n1  SetiL0=off  InitialCurrent=0  Capacitance=0  Setx0=off  InitialVoltage=0  Measurements=None
  Series RLC Branch11 : spsSeriesRLCBranchLib/Series RLC Branch  LConnTagsString=__new0  RConnTagsString=__new0  BranchType=RL  Resistance=Rg_n1  Inductance=Lg_n1  SetiL0=off  InitialCurrent=0  Capacitance=0  Setx0=off  InitialVoltage=0  Measurements=None
  Series RLC Branch2 : spsSeriesRLCBranchLib/Series RLC Branch  LConnTagsString=__new0  RConnTagsString=__new0  BranchType=RL  Resistance=Rg_n2  Inductance=Lg_n2  SetiL0=off  InitialCurrent=0  Capacitance=0  Setx0=off  InitialVoltage=0  Measurements=None
  Series RLC Branch3 : spsSeriesRLCBranchLib/Series RLC Branch  LConnTagsString=__new0  RConnTagsString=__new0  BranchType=RL  Resistance=Rg_n2  Inductance=Lg_n2  SetiL0=off  InitialCurrent=0  Capacitance=0  Setx0=off  InitialVoltage=0  Measurements=None
  Series RLC Branch9 : spsSeriesRLCBranchLib/Series RLC Branch  LConnTagsString=__new0  RConnTagsString=__new0  BranchType=RL  Resistance=Rg_n1  Inductance=Lg_n1  SetiL0=off  InitialCurrent=0  Capacitance=0  Setx0=off  InitialVoltage=0  Measurements=None
  a : PMIOPort  Side=Right
  b : PMIOPort  Port=2  Side=Right
  c : PMIOPort  Port=3  Side=Right
  vg_abc_n1 : Outport
  grid_angle : Outport  Port=2
  wires:
  Mux5/1 -> vg_abc_n1/1
  Grid/1(vza) -> Mux5/1, Controlled Voltage Source3/1
  Grid/2(vzb) -> Controlled Voltage Source4/1, Mux5/2
  Grid/3(vzc) -> Mux5/3, Controlled Voltage Source5/1
  voltage_grid/1 -> Grid/2(voltage_grid)
  Omega_grid/1 -> Grid/1(Omega_grid)
  angle_grid/1 -> Grid/3(angle_grid)
  Grid/4(grid_angle) -> grid_angle/1
  connections:
  Controlled Voltage Source3/LConn1 -- Ground/LConn1 -- Controlled Voltage Source5/LConn1 -- Controlled Voltage Source4/LConn1
  Controlled Voltage Source3/RConn1 -- Series RLC Branch3/LConn1 -- Series RLC Branch9/LConn1
  a/RConn1 -- Series RLC Branch3/RConn1 -- Series RLC Branch9/RConn1
  Controlled Voltage Source4/RConn1 -- Series RLC Branch1/LConn1 -- Series RLC Branch10/LConn1
  c/RConn1 -- Series RLC Branch2/RConn1 -- Series RLC Branch11/RConn1
  Controlled Voltage Source5/RConn1 -- Series RLC Branch2/LConn1 -- Series RLC Branch11/LConn1
  b/RConn1 -- Series RLC Branch1/RConn1 -- Series RLC Branch10/RConn1
